simulink model "scheme1"  (R2021a)
settings: Solver=FixedStepAuto  StartTime=0.0  StopTime=20  FixedStep=Tp  RelTol=1e-3
values from neighbouring files (symbols this model uses):
  k = 6    [exercise4.m]
  kp = 1.6    [exercise4.m]
  T_1 = 5.9    [exercise4.m]
  T_2 = 0.8    [exercise4.m]
  Td = 0.08    [exercise4.m]
  Ti = 6    [exercise4.m]
settings Model: Creator=Paweł  LastModifiedBy=Paweł

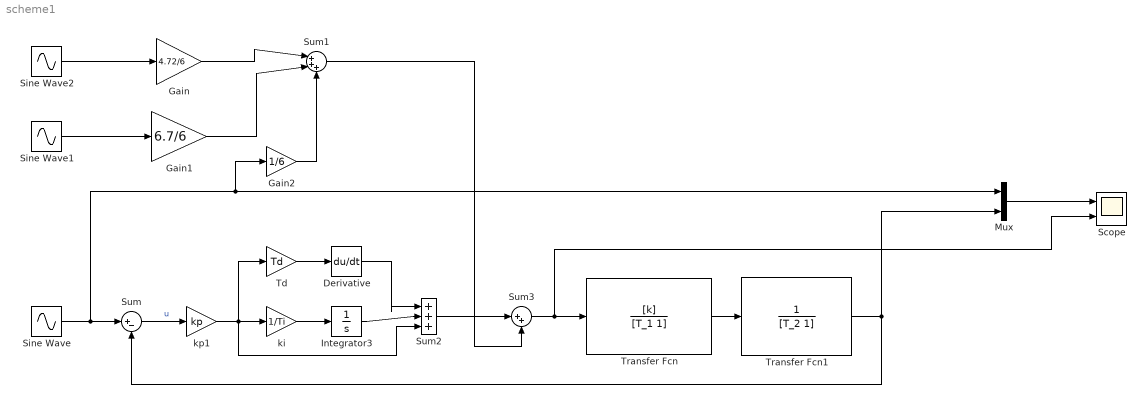
== system scheme1 ==
  Derivative : Derivative
  Gain : Gain  Gain=4.72/6
  Gain1 : Gain  Gain=6.7/6
  Gain2 : Gain  Gain=1/6
  Integrator3 : Integrator
  Mux : Mux  Inputs=2
  Scope : Scope  NumInputPorts=2
  Sine Wave : Sin  Frequency=2  SampleTime=0
  Sine Wave1 : Sin  Amplitude=2  Frequency=2  Phase=pi/2  SampleTime=0
  Sine Wave2 : Sin  Amplitude=-4  Frequency=2  SampleTime=0
  Sum : Sum  Inputs=|+-
  Sum1 : Sum  Inputs=|+++
  Sum2 : Sum  Inputs=|+++  SaturateOnIntegerOverflow=on
  Sum3 : Sum  Inputs=|++
  Td : Gain  Gain=Td  SaturateOnIntegerOverflow=on  OutDataTypeStr=Inherit: Same as input  ParamDataTypeStr=Inherit: Same as input
  Transfer Fcn : TransferFcn  Numerator=[k]  Denominator=[T_1 1]
  Transfer Fcn1 : TransferFcn  Denominator=[T_2 1]
  ki : Gain  Gain=1/Ti  SaturateOnIntegerOverflow=on  OutDataTypeStr=Inherit: Same as input  ParamDataTypeStr=Inherit: Same as input
  kp1 : Gain  Gain=kp  SaturateOnIntegerOverflow=on  OutDataTypeStr=Inherit: Same as input  ParamDataTypeStr=Inherit: Same as input
  wires:
  kp1/1 -> Td/1, Sum2/3, ki/1
  Td/1 -> Derivative/1
  Transfer Fcn/1 -> Transfer Fcn1/1
  ki/1 -> Integrator3/1
  Sine Wave/1 -> Gain2/1, Mux/1, Sum/1
  Integrator3/1 -> Sum2/2
  Derivative/1 -> Sum2/1
  Transfer Fcn1/1 -> Sum/2, Mux/2
  Sum/1 -> kp1/1  "u"
  Sine Wave2/1 -> Gain/1
  Sine Wave1/1 -> Gain1/1
  Gain/1 -> Sum1/1
  Gain1/1 -> Sum1/2
  Sum3/1 -> Scope/2, Transfer Fcn/1
  Sum2/1 -> Sum3/1
  Sum1/1 -> Sum3/2
  Gain2/1 -> Sum1/3
  Mux/1 -> Scope/1
